simulink model "Assignment_4"  (R2021a)
settings: Solver=VariableStepAuto  StartTime=0.0  StopTime=100  RelTol=1e-3
undefined symbols (not defined in the file): A, B, C1, K
libraries: simulink x1
settings Model: Creator=Tushar  LastModifiedBy=Tushar

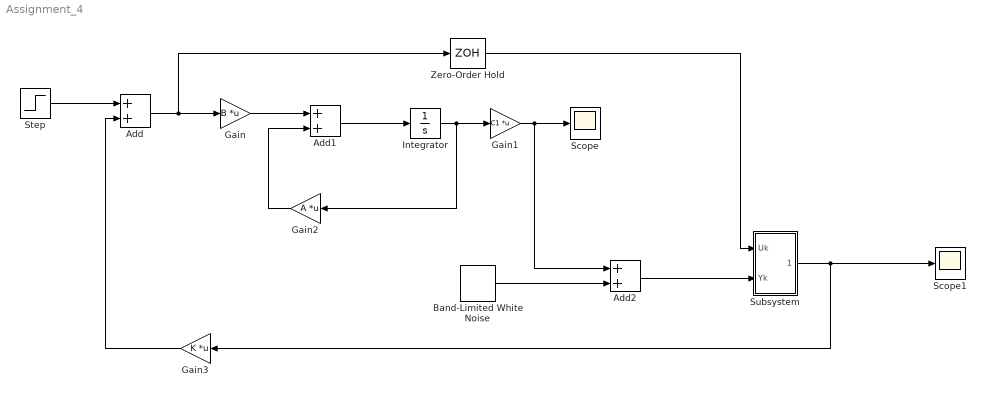
== system Assignment_4 ==
  Add : Sum
  Add1 : Sum
  Add2 : Sum
  Band-Limited White Noise : simulink/Sources/Band-Limited White Noise  Cov=0.005  Ts=0.1  seed=[23341]
  Gain : Gain  Gain=B  Multiplication=Matrix(K*u)
  Gain1 : Gain  Gain=C1  Multiplication=Matrix(K*u)
  Gain2 : Gain  Gain=A  Multiplication=Matrix(K*u)
  Gain3 : Gain  Gain=K  Multiplication=Matrix(K*u)
  Integrator : Integrator  InitialCondition=[0; 0.17; 0; 0]
  Scope : Scope
  Scope1 : Scope
  Step : Step  Time=0  SampleTime=0
  Subsystem : Subsystem
  Zero-Order Hold : ZeroOrderHold  SampleTime=-1
  wires:
  Gain/1 -> Add1/1
  Add1/1 -> Integrator/1
  Integrator/1 -> Gain2/1, Gain1/1
  Gain2/1 -> Add1/2
  Gain1/1 -> Add2/1, Scope/1
  Band-Limited White Noise/1 -> Add2/2
  Subsystem/1(Out1) -> Scope1/1, Gain3/1
  Add/1 -> Zero-Order Hold/1, Gain/1
  Add2/1 -> Subsystem/2(Yk)
  Gain3/1 -> Add/2
  Step/1 -> Add/1
  Zero-Order Hold/1 -> Subsystem/1(Uk)

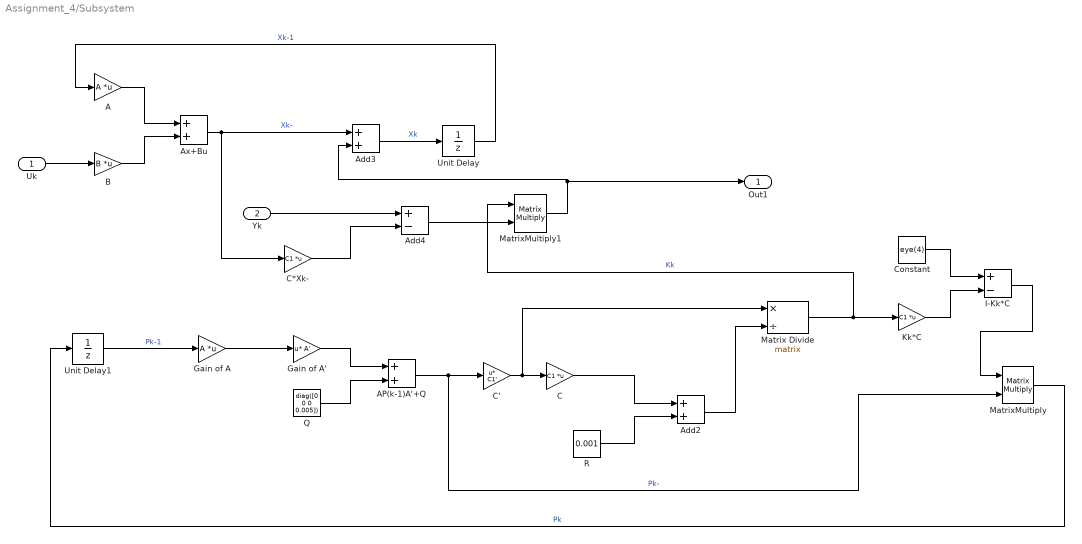
== system Assignment_4/Subsystem ==
  Uk : Inport
  Yk : Inport  Port=2
  A : Gain  Gain=A  Multiplication=Matrix(K*u)
  AP(k-1)A'+Q : Sum
  Add2 : Sum
  Add3 : Sum
  Add4 : Sum  Inputs=+-
  Ax+Bu : Sum
  B : Gain  Gain=B  Multiplication=Matrix(K*u)
  C : Gain  Gain=C1  Multiplication=Matrix(K*u)
  C' : Gain  Gain=C1'  Multiplication=Matrix(u*K)
  C*Xk- : Gain  Gain=C1  Multiplication=Matrix(K*u)
  Constant : Constant  Value=eye(4)
  Gain of A : Gain  Gain=A  Multiplication=Matrix(K*u)
  Gain of A' : Gain  Gain=A'  Multiplication=Matrix(u*K)
  I-Kk*C : Sum  Inputs=+-
  Kk*C : Gain  Gain=C1  Multiplication=Matrix(K*u)
  Matrix Divide : Product  Inputs=*/  Multiplication=Matrix(*)
  MatrixMultiply : Product  Multiplication=Matrix(*)
  MatrixMultiply1 : Product  Multiplication=Matrix(*)
  Q : Constant  Value=diag([0 0 0 0.005])
  R : Constant  Value=0.001
  Unit Delay : UnitDelay  SampleTime=-1  HasFrameUpgradeWarning=on
  Unit Delay1 : UnitDelay  SampleTime=-1  HasFrameUpgradeWarning=on
  Out1 : Outport
  wires:
  AP(k-1)A'+Q/1 -> MatrixMultiply/2, C'/1  "Pk-"
  Matrix Divide/1 -> MatrixMultiply1/1, Kk*C/1  "Kk"
  B/1 -> Ax+Bu/2
  Yk/1 -> Add4/1
  Unit Delay/1 -> A/1  "Xk-1"
  Add3/1 -> Unit Delay/1  "Xk"
  Kk*C/1 -> I-Kk*C/2
  Ax+Bu/1 -> C*Xk-/1, Add3/1  "Xk-"
  Gain of A/1 -> Gain of A'/1
  Constant/1 -> I-Kk*C/1
  Gain of A'/1 -> AP(k-1)A'+Q/1
  A/1 -> Ax+Bu/1
  MatrixMultiply1/1 -> Add3/2, Out1/1
  Add2/1 -> Matrix Divide/2
  C'/1 -> Matrix Divide/1, C/1
  C/1 -> Add2/1
  Add4/1 -> MatrixMultiply1/2
  C*Xk-/1 -> Add4/2
  I-Kk*C/1 -> MatrixMultiply/1
  Q/1 -> AP(k-1)A'+Q/2
  R/1 -> Add2/2
  MatrixMultiply/1 -> Unit Delay1/1  "Pk"
  Unit Delay1/1 -> Gain of A/1  "Pk-1"
  Uk/1 -> B/1
